simulink model "quad_with_sensor_fusion"  (R2022b)
settings: Solver=ode4  StartTime=0.0  StopTime=120  FixedStep=0.005  RelTol=1e-3
values from neighbouring files (symbols this model uses):
  Ixc = 9373.661914436/1e6    (= 0.00937366191444)    [ParamsInit_test.m]
  Iyc = 11755.067703159/1e6    (= 0.0117550677032)    [ParamsInit_test.m]
  Izc = 17533.553367555/1e6    (= 0.0175335533676)    [ParamsInit_test.m]
  kd_h = damp_ratio_h*2*sqrt(kp_h*Vehicle.Airframe.mass)    [ParamsInit_test.m]
  kd_phi = damp_ratio_phi*2*sqrt(kp_phi*Ixc)    [ParamsInit_test.m]
  kd_theta = damp_ratio_theta*2*sqrt(kp_theta*Iyc)    [ParamsInit_test.m]
  kd_yaw = damp_ratio_yaw*2*sqrt(kp_yaw*Izc)    [ParamsInit_test.m]
  kp_h = omega_n_h^2*Vehicle.Airframe.mass    [ParamsInit_test.m]
  kp_phi = omega_n_phi^2*Ixc    (= 0.937366191444)    [ParamsInit_test.m]
  kp_position = 0.1    [ParamsInit_test.m]
  kp_theta = omega_n_theta^2*Iyc    (= 1.17550677032)    [ParamsInit_test.m]
  kp_vx = 0.25    [ParamsInit_test.m]
  kp_vy = 0.25    [ParamsInit_test.m]
  kp_yaw = omega_n_yaw^2*Izc    (= 0.0175335533676)    [ParamsInit_test.m]
undefined symbols (not defined in the file or in its folder): Vehicle
libraries: simulink x3, aerolibconvert2 x2, mspfiltlib x1, sensorinslib x1, aerolibasang x1, sharedtransform x1, aerolibanimutils x1, uavutilslib x1
(part 2 of 2)

== matlab function quad_with_sensor_fusion/Sensors and Sensor Fusion/Subsystem6/MATLAB Function1 ==
  data: thetadot output; Q input; R input; phi input
function thetadot = fcn(Q,R,phi)
    thetadot = cos(phi)*Q-sin(phi)*R;
end

== matlab function quad_with_sensor_fusion/Sensors and Sensor Fusion/Subsystem6/MATLAB Function2 ==
  data: pusaidot output; Q input; R input; phi input; theta input
function pusaidot = fcn(Q,R,phi,theta)
    pusaidot = sin(phi)*sec(theta)*Q+cos(phi)*sec(theta)*R;
end
